simulink model "PMSM_to_BLDC_mod1"  (R2025b)
settings: Solver=FixedStepAuto  StartTime=0.0  StopTime=100  FixedStep=0.001  RelTol=1e-3
values from neighbouring files (symbols this model uses):
  B = 0.0025    [PMSM_to_BLDC_FOC.m]
  ctrl_reg1 = 0x02    [PMSM_to_BLDC_FOC.m]
  ctrl_reg2 = 0x03    [PMSM_to_BLDC_FOC.m]
  Damping_viscous = 0.00012    [PMSM_to_BLDC_FOC.m]
  J = 4.5e-5    (= 4.5e-05)    [PMSM_to_BLDC_FOC.m]
  Ki_Id = omg_clc * R_s    (= 464.72)    [PMSM_to_BLDC_FOC.m]
  Ki_Iq = omg_clc * R_s    (= 464.72)    [PMSM_to_BLDC_FOC.m]
  ki_speed = ((B *omg_cls * omg_cls)/(1.5*motor_polepairs*flux_linkage))    (= 157373.358662)    [PMSM_to_BLDC_FOC.m]
  Kp_Id = omg_clc * Ld    (= 22.608)    [PMSM_to_BLDC_FOC.m]
  Kp_Iq = omg_clc * Lq    (= 22.608)    [PMSM_to_BLDC_FOC.m]
  kp_speed = ((J*omg_cls)/(1.5*motor_polepairs*flux_linkage))    (= 2.25535068146)    [PMSM_to_BLDC_FOC.m]
  motor_polepairs = 7    [PMSM_to_BLDC_FOC.m]
  pwm_frequency = 20e3    (= 20000)    [PMSM_to_BLDC_FOC.m]
  read_reg = 1    [PMSM_to_BLDC_FOC.m]
  reg_ctrl_2 = ( bitshift(0,6) + bitshift(0,4) + bitshift(1,2) + bitshift(0,0))    [PMSM_to_BLDC_FOC.m]
  rps = x/6.28    (= 15.923566879)    [PMSM_to_BLDC_FOC.m]
  stat_reg1 = 0x00    [PMSM_to_BLDC_FOC.m]
  stat_reg2 = 0x01    [PMSM_to_BLDC_FOC.m]
  write_reg = 0    [PMSM_to_BLDC_FOC.m]
  x = 100    [PMSM_to_BLDC_FOC.m]
libraries: stm32blockslib x14, simulink x12, hdlsllib x10, nesl_utility x9, stm32f4xxblockslib x5, slpidlib x5, fl_lib x5, mcbeeMathTransformLib x3, ee_lib x3, mcbcontrolslib x1, mcbsensorlessestimatorlib x1, mcbplantlib x1
(part 1 of 2)
settings Model: STM32="{\"AnalogInput\":[{\"ID\":\"PMSM_to_BLDC_mod1:630\"},{\"ID\":\"PMSM_to_BLDC_mod1:900\"},{\"ID\":\"PMSM_to_BLDC_mod1:904\"}],\"PWMOutput\":{\"ID\":\"PMSM_to_BLDC_mod1:632\"},\"SPIControllerTransfer\":[{\"ID\":\"PMSM_to_BLDC_mod1:1052\"},{\"ID\":\"PMSM_to_BLDC_mod1:1051\"},{\"ID\":\"PMSM_to_BLDC_mod1:1149\"}],\"SPIControllerTransmit\":[{\"ID\":\"PMSM_to_BLDC_mod1:1060\"},{\"ID\":\"PMSM_to_BLDC_mod1:636:1184\"},{\"ID\":\"PMSM_to_BLDC_mod1:1221\"},{\"ID\":\"PMSM_to_BLDC_mod1:1178:1430\"},{\"ID\":\"PMSM_to_BLDC_mod1:1458\"},{\"ID\":\"PMSM_to_BLDC_mod1:1472\"},{\"ID\":\"PMSM_to_BLDC_mod1:1612\"},{\"ID\":\"PMSM_to_BLDC_mod1:1438\"},{\"ID\":\"PMSM_to_BLDC_mod1:1637\"},{\"ID\":\"PMSM_to_BLDC_mod1:1643\"}],\"DigitalPortWrite\":[{\"ID\":\"PMSM_to_BLDC_mod1:672\"},{\"ID\":\"PMSM_to_BLDC_mod1:1183\"}],\"SPIControllerReceive\":[{\"ID\":\"PMSM_to_BLDC_mod1:1178:1431\"},{\"ID\":\"PMSM_to_BLDC_mod1:1431\"},{\"ID\":\"PMSM_to_BLDC_mod1:1457\"},{\"ID\":\"PMSM_to_BLDC_mod1:1471\"},{\"ID\":\"PMSM_to_BLDC_mod1:1614\"},{\"ID\":\"PMSM_to_BLDC_mod1:1439\"},{\"ID\":\"PMSM_to_BLDC_mod1:1636\"},{\"ID\":\"PMSM_to_BLDC_mod1:1642\"}]}"  NumberOfSteps=5  Creator=Surinova  LastModifiedBy=Surinova
settings SolverCC: AutoInsertRateTranBlk=on
settings OptimizationCC: DefaultParameterBehavior=Inlined  EnhancedBackFolding=on  PassReuseOutputArgsAs=Individual arguments  ZeroExternalMemoryAtStartup=off  ZeroInternalMemoryAtStartup=off  MaxStackSize=512  OptimizeBlockOrder=speed  DifferentSizesBufferReuse=on  OptimizationCustomize=off  EfficientTunableParamExpr=on
settings DebuggingCC: ParameterTunabilityLossMsg=error
settings HardwareCC: ProdBitPerPointer=32.0  ProdBitPerSizeT=32.0  ProdBitPerPtrDiffT=32.0  ProdLargestAtomicInteger=Long  ProdLargestAtomicFloat=Double  ProdWordSize=32.0  ProdLongLongMode=on  ProdHWDeviceType=ARM Compatible->ARM Cortex-M
settings SFSimCC: SimCustomHeaderCode="\"C:\\Users\\Surinova\\OneDrive - Surinova Pvt Ltd\\Documents\\Github\\MatLab_FOC_model\\FOC_model_1\\SPI_code.h\""  SimUserSources="\"C:\\Users\\Surinova\\OneDrive - Surinova Pvt Ltd\\Documents\\Github\\MatLab_FOC_model\\FOC_model_1\\SPI_code.c\""  MATLABDynamicMemAlloc=off
settings RTWCC: SystemTargetFile=ert.tlc  HardwareBoard=STM32F4xx Based  TemplateMakefile=ert_default_tmf  GenerateReport=on  Toolchain=GNU Tools for ARM Embedded Processors  LaunchReport=on  Description=Embedded Coder
settings RTWCC: CustomHeaderCode=|
  | #include "main.h"
  | #include "SPI_code.h"
  | #include "spi.h"
  | #include "dma.h"
  | #include "gpio.h"
  | #include "tim.h"
  | #include "adc.h"
  | #include "usart.h"
settings RTWCC: CustomInclude=|
  | "C:\Users\Surinova\OneDrive - Surinova Pvt Ltd\Documents\Github\MatLab_FOC_model\FOC_model_1"
  | "C:\Users\Surinova\OneDrive - Surinova Pvt Ltd\Documents\Github\MatLab_FOC_model\F405_PMSM_Mod1\Core\Inc"
  | "C:\Users\Surinova\OneDrive - Surinova Pvt Ltd\Documents\Github\MatLab_FOC_model\F405_PMSM_Mod1\Drivers\STM32F4xx_HAL_Driver\Inc"
  | "C:\Users\Surinova\OneDrive - Surinova Pvt Ltd\Documents\Github\MatLab_FOC_model\F405_PMSM_Mod1\Drivers\CMSIS\Include"
  | "C:\Users\Surinova\OneDrive - Surinova Pvt Ltd\Documents\Github\MatLab_FOC_model\F405_PMSM_Mod1\Drivers\CMSIS\Device\ST\STM32F4xx\Include"
settings RTWCC: CustomSource=|
  | SPI_code.c
  | "C:\Users\Surinova\OneDrive - Surinova Pvt Ltd\Documents\Github\MatLab_FOC_model\F405_PMSM_Mod1\Drivers\STM32F4xx_HAL_Driver\Src\stm32f4xx_hal_spi.c"
  | "C:\Users\Surinova\OneDrive - Surinova Pvt Ltd\Documents\Github\MatLab_FOC_model\F405_PMSM_Mod1\Core\Src\spi.c"
  | "C:\Users\Surinova\OneDrive - Surinova Pvt Ltd\Documents\Github\MatLab_FOC_model\F405_PMSM_Mod1\Core\Src\adc.c"
  | "C:\Users\Surinova\OneDrive - Surinova Pvt Ltd\Documents\Github\MatLab_FOC_model\F405_PMSM_Mod1\Core\Src\dma.c"
  | "C:\Users\Surinova\OneDrive - Surinova Pvt Ltd\Documents\Github\MatLab_FOC_model\F405_PMSM_Mod1\Core\Src\gpio.c"
  | "C:\Users\Surinova\OneDrive - Surinova Pvt Ltd\Documents\Github\MatLab_FOC_model\F405_PMSM_Mod1\Core\Src\tim.c"
  | "C:\Users\Surinova\OneDrive - Surinova Pvt Ltd\Documents\Github\MatLab_FOC_model\F405_PMSM_Mod1\Core\Src\usart.c"
settings CodeAppCC: ForceParamTrailComments=on  IgnoreCustomStorageClasses=off  OperatorAnnotations=on  SimulinkDataObjDesc=on  SFDataObjDesc=on  InsertBlockDesc=on
settings ERTTargetCC: ExtModeTransport=3.0  ExtModeStaticAlloc=on  ExtModeStaticAllocSize=2048.0  ExtModeMexFile=ext_xcp  ExtModeIntrfLevel=Level2 - Open  TargetLangStandard=C99 (ISO)  CodeReplacementLibrary=ARM Cortex-M  SupportContinuousTime=on

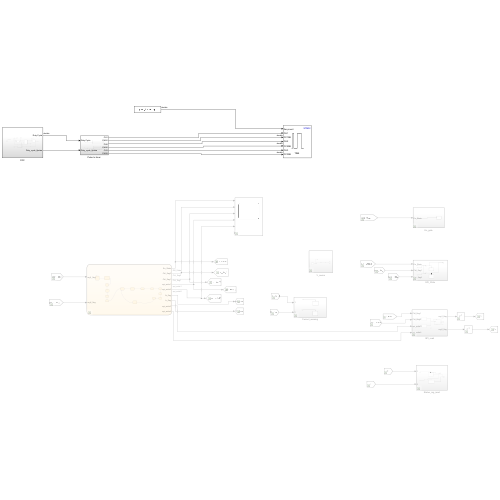
[thumbnail: Simulink's stored preview of the top-level diagram]
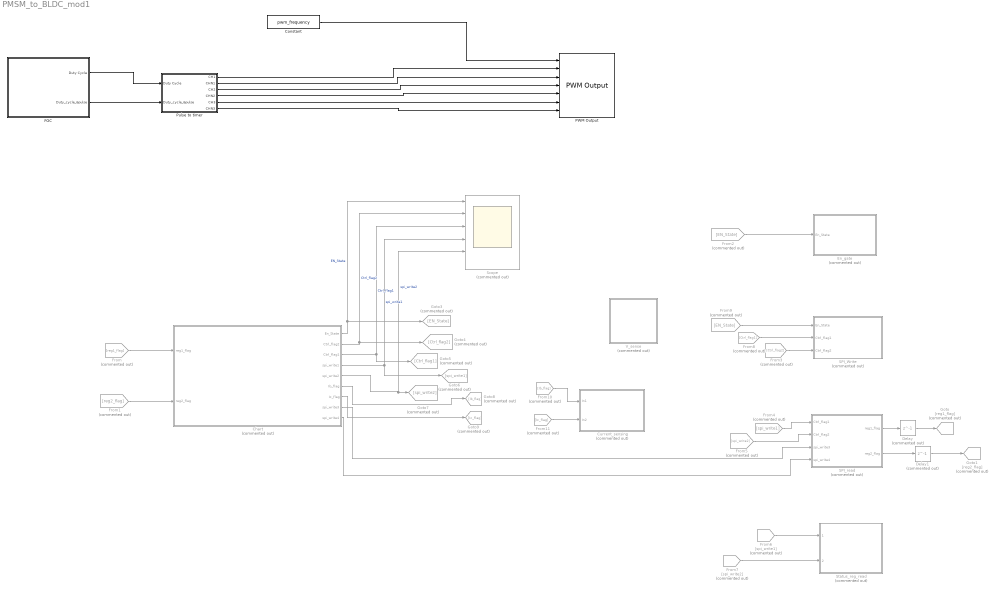
== system PMSM_to_BLDC_mod1 ==
  Chart : Stateflow chart  Commented=on  TreatAsAtomicUnit=on
  Constant : Constant  Value=pwm_frequency
  Current_sensing : Subsystem  Commented=on
  Delay : Delay  Commented=on  DelayLength=1  InputProcessing=Columns as channels (frame based)
  Delay1 : Delay  Commented=on  DelayLength=1  InputProcessing=Columns as channels (frame based)
  En_gate : Subsystem  Commented=on
  FOC : Subsystem
  From : From  Commented=on  GotoTag=reg1_flag
  From1 : From  Commented=on  GotoTag=reg2_flag
  From10 : From  Commented=on  GotoTag=Ib_flag
  From11 : From  Commented=on  GotoTag=Ic_flag
  From2 : From  Commented=on  GotoTag=EN_State
  From3 : From  Commented=on  GotoTag=Ctrl_flag2
  From4 : From  Commented=on  GotoTag=spi_write1
  From5 : From  Commented=on  GotoTag=spi_write2
  From6 : From  Commented=on  GotoTag=spi_write1
  From7 : From  Commented=on  GotoTag=spi_write2
  From8 : From  Commented=on  GotoTag=Ctrl_flag1
  From9 : From  Commented=on  GotoTag=EN_State
  Goto : Goto  Commented=on  GotoTag=reg1_flag
  Goto1 : Goto  Commented=on  GotoTag=reg2_flag
  Goto3 : Goto  Commented=on  GotoTag=EN_State
  Goto4 : Goto  Commented=on  GotoTag=Ctrl_flag2
  Goto5 : Goto  Commented=on  GotoTag=Ctrl_flag1
  Goto6 : Goto  Commented=on  GotoTag=spi_write1
  Goto7 : Goto  Commented=on  GotoTag=spi_write2
  Goto8 : Goto  Commented=on  GotoTag=Ib_flag
  Goto9 : Goto  Commented=on  GotoTag=Ic_flag
  PWM Output : stm32f4xxblockslib/PWM Output  ProcessorFamily=STM32F4  TimerModule=TIM8  DutycycleUnits=Percentage  EnableChannel1=on  EnableCaptureCompare1Input=off  EnableCaptureCompare1ComplementaryInput=on  EnableOutputCompare1ModeInput=off  EnableChannel2=on  EnableCaptureCompare2Input=off  EnableCaptureCompare2ComplementaryInput=on  EnableOutputCompare2ModeInput=off  EnableChannel3=on  EnableCaptureCompare3Input=off  EnableCaptureCompare3ComplementaryInput=on  EnableOutputCompare3ModeInput=off  EnableChannel4=off  EnableCaptureCompare4Input=off  EnableCaptureCompare4ComplementaryInput=off  EnableOutputCompare4ModeInput=off  EnableChannel5=off  EnableCaptureCompare5Input=off  EnableOutputCompare5ModeInput=off  EnableChannel6=off  EnableCaptureCompare6Input=off  EnableOutputCompare6ModeInput=off  EnableCounterInput=off  EnableMainOutputInput=off  EnableFrequencyInput=on  SetRCAfterCE=on  OutputDirection=off  OutputMainOutputEnableStatus=off  SampleTime=0.1  EnableSimPort=off  EnableUpdateEvent=off  EnableCaptureCompare1Event=off  EnableCaptureCompare2Event=off  EnableCaptureCompare3Event=off  EnableCaptureCompare4Event=off  EnableTriggerEvent=off  EnableBreakEvent=off  EnableBreakEvent2=off  hoistedMaskSrc=ECSoC/ECSimCodegen/PWM Output
  "Pulse to timer " : Subsystem
  SPI_Write : Subsystem  Commented=on
  SPI_read : Subsystem  Commented=on
  Scope : Scope  Commented=on  NumInputPorts=6
      settings: ActiveDisplayYMinimum=-0.011045533032348887  ActiveDisplayYMaximum=0.023895922034976431  DataLoggingVariableName=ScopeData17
  Status_reg_read : Subsystem  Commented=on
  V_sense : Subsystem  Commented=on
  wires:
  Constant/1 -> PWM Output/1
  FOC/1(Duty Cycle) -> "Pulse to timer "/1(Duty Cycle)
  SPI_read/1(reg1_flag) -> Delay/1
  SPI_read/2(reg2_flag) -> Delay1/1
  From/1 -> Chart/1(reg1_flag)
  From1/1 -> Chart/2(reg2_flag)
  Chart/1(En_State) -> Scope/1, Goto3/1  "EN_State"
  Chart/2(Ctrl_flag2) -> Goto4/1, Scope/2  "Ctrl_flag2"
  Chart/3(Ctrl_flag1) -> Goto5/1, Scope/3  "Ctrl_flag1"
  Chart/4(spi_write1) -> Goto6/1, Scope/4  "spi_write1"
  Chart/5(spi_write2) -> Goto7/1, Scope/5  "spi_write2"
  Chart/6(Ib_flag) -> Goto8/1
  Chart/7(Ic_flag) -> Goto9/1
  From2/1 -> En_gate/1(En_State)
  From9/1 -> SPI_Write/1(En_State)
  From8/1 -> SPI_Write/2(Ctrl_flag1)
  From4/1 -> SPI_read/1(Ctrl_flag1)
  From5/1 -> SPI_read/2(Ctrl_flag2)
  From6/1 -> Status_reg_read/1(1)
  From7/1 -> Status_reg_read/2(2)
  From10/1 -> Current_sensing/1(In1)
  From11/1 -> Current_sensing/2(In2)
  From3/1 -> SPI_Write/3(Ctrl_flag2)
  Chart/8(spi_write3) -> SPI_read/3(spi_write3)
  Chart/9(spi_write4) -> SPI_read/4(spi_write4)
  Delay/1 -> Goto/1
  Delay1/1 -> Goto1/1
  FOC/2(Duty_cycle_6pulse) -> "Pulse to timer "/2(Duty_cycle_6pulse)
  "Pulse to timer "/1(CH1) -> PWM Output/2
  "Pulse to timer "/2(CHN1) -> PWM Output/3
  "Pulse to timer "/3(CH2) -> PWM Output/4
  "Pulse to timer "/4(CHN2) -> PWM Output/5
  "Pulse to timer "/5(CH3) -> PWM Output/6
  "Pulse to timer "/6(CHN3) -> PWM Output/7

== system PMSM_to_BLDC_mod1/Current_sensing ==
  In1 : Inport
  In2 : Inport  Port=2
  Subsystem : Subsystem
  Subsystem1 : Subsystem
  wires:
  In1/1 -> Subsystem/Enable
  In2/1 -> Subsystem1/Enable

== system PMSM_to_BLDC_mod1/En_gate ==
  En_State : Inport
  Digital Port Write : stm32f4xxblockslib/Digital Port Write  PortName=GPIOB  PinNumber=12  ReadOperation=off  IOAsArray=on  EnableSimPort=off  hoistedMaskSrc=ECSoC/ECSimCodegen/Digital Port Write
  wires:
  En_State/1 -> Digital Port Write/1

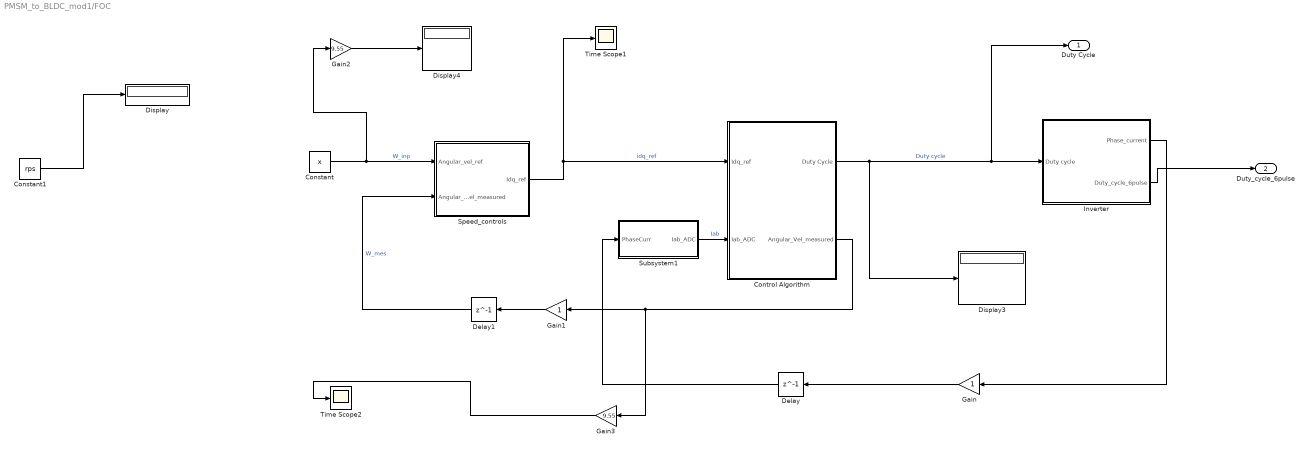
== system PMSM_to_BLDC_mod1/FOC ==
  Constant : Constant  Value=x
  Constant1 : Constant  Value=rps
  "Control Algorithm " : Subsystem
  Delay : Delay  DelayLength=1
  Delay1 : Delay  DelayLength=1
  Display : Display
  Display3 : Display
  Display4 : Display
  Gain : Gain
  Gain1 : Gain
  Gain2 : Gain  Gain=9.55
  Gain3 : Gain  Gain=9.55
  Inverter : Subsystem
  Speed_controls : Subsystem
  Subsystem1 : Subsystem
  Time Scope1 : Scope
      settings: TimeUnits=Metric (based on Time Span)  ActiveDisplayYMinimum=-1278.396312713623  ActiveDisplayYMaximum=607.25992965698242  YLabel=Amplitude
  Time Scope2 : Scope
      settings: TimeUnits=Metric (based on Time Span)  ActiveDisplayYMinimum=-2551.3535904439232  ActiveDisplayYMaximum=7986.0366937033405  YLabel=Amplitude  DataLoggingVariableName=ScopeData5
  Duty Cycle : Outport
  Duty_cycle_6pulse : Outport  Port=2
  wires:
  Delay1/1 -> Speed_controls/2(Angular_vel_measured)  "W_mes"
  Subsystem1/1(Iab_ADC) -> "Control Algorithm "/2(Iab_ADC)  "Iab"
  Gain3/1 -> Time Scope2/1
  Constant/1 -> Gain2/1, Speed_controls/1(Angular_vel_ref)  "W_inp"
  Gain/1 -> Delay/1
  "Control Algorithm "/2(Angular_Vel_measured) -> Gain1/1, Gain3/1
  Gain2/1 -> Display4/1
  "Control Algorithm "/1(Duty Cycle) -> Duty Cycle/1, Inverter/1(Duty cycle), Display3/1  "Duty cycle"
  Constant1/1 -> Display/1
  Speed_controls/1(Idq_ref) -> Time Scope1/1, "Control Algorithm "/1(Idq_ref)  "idq_ref"
  Gain1/1 -> Delay1/1
  Inverter/1(Phase_current) -> Gain/1
  Delay/1 -> Subsystem1/1(PhaseCurr)
  Inverter/2(Duty_cycle_6pulse) -> Duty_cycle_6pulse/1

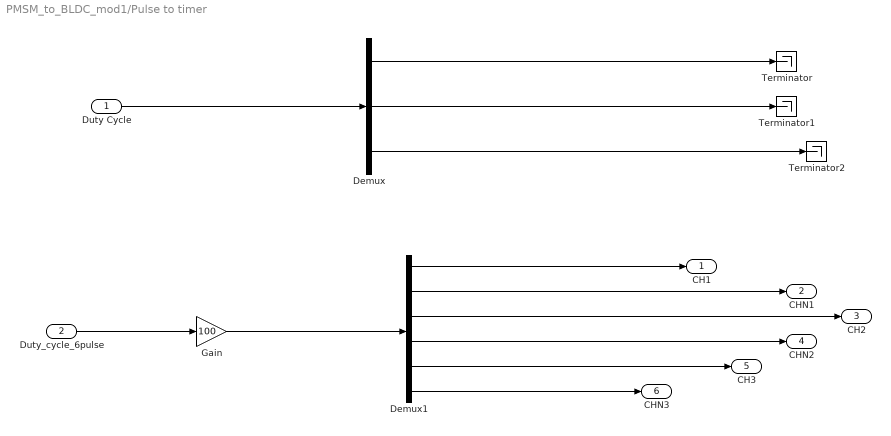
== system PMSM_to_BLDC_mod1/Pulse to timer  ==
  Duty Cycle : Inport
  Duty_cycle_6pulse : Inport  Port=2
  Demux : Demux  Outputs=3
  Demux1 : Demux  Outputs=6
  Gain : Gain  Gain=100
  Terminator : Terminator
  Terminator1 : Terminator
  Terminator2 : Terminator
  CH1 : Outport
  CHN1 : Outport  Port=2
  CH2 : Outport  Port=3
  CHN2 : Outport  Port=4
  CH3 : Outport  Port=5
  CHN3 : Outport  Port=6
  wires:
  Duty Cycle/1 -> Demux/1
  Demux/3 -> Terminator2/1
  Demux/1 -> Terminator/1
  Demux/2 -> Terminator1/1
  Duty_cycle_6pulse/1 -> Gain/1
  Demux1/1 -> CH1/1
  Demux1/2 -> CHN1/1
  Demux1/3 -> CH2/1
  Demux1/4 -> CHN2/1
  Demux1/5 -> CH3/1
  Demux1/6 -> CHN3/1
  Gain/1 -> Demux1/1

== system PMSM_to_BLDC_mod1/SPI_Write ==
  En_State : Inport
  Ctrl_flag1 : Inport  Port=2
  Ctrl_flag2 : Inport  Port=3
  AND : Logic  IconShape=distinctive  AllPortsSameDT=off  OutDataTypeStr=boolean
  AND1 : Logic  IconShape=distinctive  AllPortsSameDT=off  OutDataTypeStr=boolean
  Control_Reg2 : Subsystem
  Ctrl_Reg_1 : Subsystem  ReferencedSubsystem=Ctrl_Reg_1
  Scope : Scope  NumInputPorts=2
      settings: ActiveDisplayYMinimum=-0.12499999999999997  ActiveDisplayYMaximum=1.125  DataLoggingVariableName=ScopeData18
  wires:
  Ctrl_flag1/1 -> AND/2
  En_State/1 -> AND1/1, AND/1
  AND/1 -> Scope/1, Ctrl_Reg_1/Enable
  AND1/1 -> Control_Reg2/Enable, Scope/2
  Ctrl_flag2/1 -> AND1/2

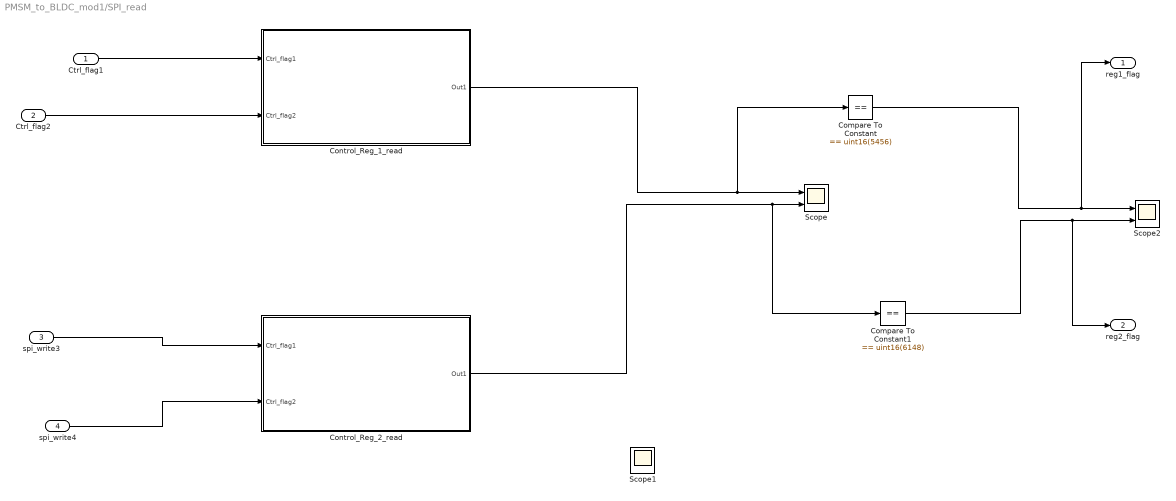
== system PMSM_to_BLDC_mod1/SPI_read ==
  Ctrl_flag1 : Inport
  Ctrl_flag2 : Inport  Port=2
  spi_write3 : Inport  Port=3
  spi_write4 : Inport  Port=4
  Compare To Constant : simulink/Logic and Bit Operations/Compare To Constant  relop===  const=uint16(5456)  OutDataTypeStr=boolean
  Compare To Constant1 : simulink/Logic and Bit Operations/Compare To Constant  relop===  const=uint16(6148)  OutDataTypeStr=boolean
  Control_Reg_1_read : Subsystem
  Control_Reg_2_read : Subsystem
  Scope : Scope  NumInputPorts=2
      settings: ActiveDisplayYMinimum=-4607.9999999999991  ActiveDisplayYMaximum=41472  DataLoggingVariableName=ScopeData13
  Scope1 : Scope  NumInputPorts=2
      settings: ActiveDisplayYMinimum=-0.082255061291701556  ActiveDisplayYMaximum=0.18007764693489475  DataLoggingVariableName=ScopeData21
  Scope2 : Scope  NumInputPorts=2
      settings: ActiveDisplayYMinimum=-0.12499999999999997  ActiveDisplayYMaximum=1.125  DataLoggingVariableName=ScopeData15
  reg1_flag : Outport
  reg2_flag : Outport  Port=2
  wires:
  Compare To Constant/1 -> reg1_flag/1, Scope2/1
  Ctrl_flag1/1 -> Control_Reg_1_read/1(Ctrl_flag1)
  Ctrl_flag2/1 -> Control_Reg_1_read/2(Ctrl_flag2)
  spi_write3/1 -> Control_Reg_2_read/1(Ctrl_flag1)
  spi_write4/1 -> Control_Reg_2_read/2(Ctrl_flag2)
  Control_Reg_1_read/1(Out1) -> Compare To Constant/1, Scope/1
  Control_Reg_2_read/1(Out1) -> Compare To Constant1/1, Scope/2
  Compare To Constant1/1 -> reg2_flag/1, Scope2/2

== system PMSM_to_BLDC_mod1/Status_reg_read ==
  1 : Inport
  2 : Inport  Port=2
  Scope : Scope  NumInputPorts=2
      settings: ActiveDisplayYMinimum=-1.2810969274237476  ActiveDisplayYMaximum=1.2714661975762531  DataLoggingVariableName=ScopeData14
  Scope1 : Scope  NumInputPorts=2
      settings: ActiveDisplayYMinimum=-1.7236670282456201  ActiveDisplayYMaximum=2.8116607909152096  DataLoggingVariableName=ScopeData16
  Status_Reg1_read : Subsystem
  Status_Reg_2_read : Subsystem
  wires:
  1/1 -> Scope1/1, Status_Reg1_read/Enable
  Status_Reg1_read/1(Out1) -> Scope/2
  Status_Reg_2_read/1(Out1) -> Scope/1
  2/1 -> Scope1/2, Status_Reg_2_read/Enable

== system PMSM_to_BLDC_mod1/V_sense ==
  Analog to Digital Converter1 : stm32f4xxblockslib/Analog to Digital Converter  ADCModule=ADC1  ConversionGroup=Regular  TriggerMode=Trigger and read  NumberOfConversions=1  EnableBufferConv=off  BufferLength=1  OutputStatus=off  SampleTime=0.1  EnableSimPort=off  hoistedMaskSrc=ECSoC/ECSimCodegen/Analog to Digital Converter
  Data Type Conversion : DataTypeConversion  OutDataTypeStr=double  SaturateOnIntegerOverflow=off  RndMeth=Floor
  Display : Display
  Gain : Gain  Gain=50/3200
  Scope : Scope
      settings: ActiveDisplayYMinimum=1998.2131563180828  ActiveDisplayYMaximum=2530.7206563180825  DataLoggingVariableName=ScopeData12
  wires:
  Analog to Digital Converter1/1 -> Scope/1, Data Type Conversion/1
  Gain/1 -> Display/1
  Data Type Conversion/1 -> Gain/1

== system PMSM_to_BLDC_mod1/Current_sensing/Subsystem ==
  Enable : EnablePort
  Analog to Digital Converter1 : stm32f4xxblockslib/Analog to Digital Converter  ADCModule=ADC2  ConversionGroup=Regular  TriggerMode=Trigger and read  NumberOfConversions=1  EnableBufferConv=off  BufferLength=1  OutputStatus=off  SampleTime=0.1  EnableSimPort=off  hoistedMaskSrc=ECSoC/ECSimCodegen/Analog to Digital Converter
  Data Type Conversion : DataTypeConversion  OutDataTypeStr=double  SaturateOnIntegerOverflow=off  RndMeth=Floor
  Display1 : Display
  Gain : Gain  Gain=100/4095
  wires:
  Gain/1 -> Display1/1
  Analog to Digital Converter1/1 -> Data Type Conversion/1
  Data Type Conversion/1 -> Gain/1

== system PMSM_to_BLDC_mod1/Current_sensing/Subsystem1 ==
  Enable : EnablePort
  Analog to Digital Converter2 : stm32f4xxblockslib/Analog to Digital Converter  ADCModule=ADC3  ConversionGroup=Regular  TriggerMode=Trigger and read  NumberOfConversions=1  EnableBufferConv=off  BufferLength=1  OutputStatus=off  SampleTime=0.1  EnableSimPort=off  hoistedMaskSrc=ECSoC/ECSimCodegen/Analog to Digital Converter
  Data Type Conversion1 : DataTypeConversion  OutDataTypeStr=double  SaturateOnIntegerOverflow=off  RndMeth=Floor
  Display2 : Display
  Gain1 : Gain  Gain=100/4095
  wires:
  Gain1/1 -> Display2/1
  Analog to Digital Converter2/1 -> Data Type Conversion1/1
  Data Type Conversion1/1 -> Gain1/1

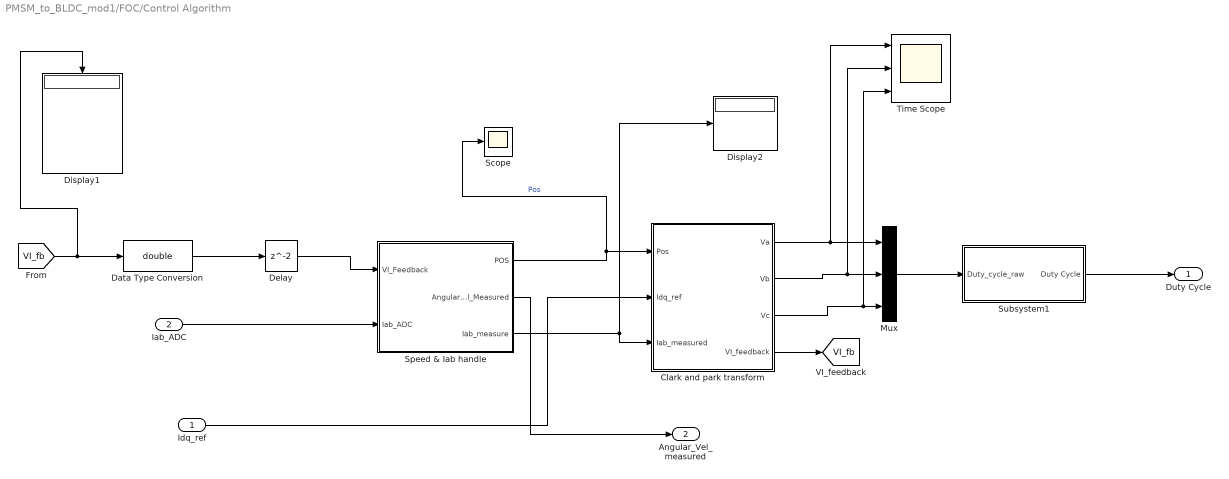
== system PMSM_to_BLDC_mod1/FOC/Control Algorithm  ==
  Idq_ref : Inport
  Iab_ADC : Inport  Port=2
  Clark and park transform : Subsystem
  Data Type Conversion : DataTypeConversion  OutDataTypeStr=double  SaturateOnIntegerOverflow=off  RndMeth=Floor
  Delay : Delay
  Display1 : Display
  Display2 : Display
  Mux : Mux  Inputs=3
  Scope : Scope
      settings: ActiveDisplayYMinimum=-2.9858848726720835  ActiveDisplayYMaximum=10.141823403799465  DataLoggingVariableName=ScopeData4
  Speed & Iab handle : Subsystem
  Subsystem1 : Subsystem
  Time Scope : Scope  NumInputPorts=3
      settings: TimeUnits=Metric (based on Time Span)  ActiveDisplayYMinimum=-4.3489349004753368  ActiveDisplayYMaximum=5.723501707770442  YLabel=Amplitude  DataLoggingVariableName=ScopeData2
  Duty Cycle : Outport
  Angular_Vel_measured : Outport  Port=2
  tag scope: VI_fb=global
  wires:
  Clark and park transform/4(VI_feedback) -> [VI_fb]
  Clark and park transform/3(Vc) -> Mux/3, Time Scope/3
  [VI_fb] -> Display1/1, Data Type Conversion/1
  Mux/1 -> Subsystem1/1(Duty_cycle_raw)
  Iab_ADC/1 -> Speed & Iab handle/2(Iab_ADC)
  Speed & Iab handle/3(Iab_measure) -> Clark and park transform/3(Iab_measured), Display2/1
  Clark and park transform/2(Vb) -> Mux/2, Time Scope/2
  Clark and park transform/1(Va) -> Time Scope/1, Mux/1
  Speed & Iab handle/2(Angular_Vel_Measured) -> Angular_Vel_measured/1
  Idq_ref/1 -> Clark and park transform/2(Idq_ref)
  Delay/1 -> Speed & Iab handle/1(VI_Feedback)
  Data Type Conversion/1 -> Delay/1
  Speed & Iab handle/1(POS) -> Scope/1, Clark and park transform/1(Pos)  "Pos"
  Subsystem1/1(Duty Cycle) -> Duty Cycle/1

== system PMSM_to_BLDC_mod1/FOC/Inverter ==
  Duty cycle : Inport
  Simulation : Subsystem
  Subsystem2 : Subsystem
  Phase_current : Outport
  Duty_cycle_6pulse : Outport  Port=2
  wires:
  Duty cycle/1 -> Simulation/2(Duty_cycle), Subsystem2/1(Duty cycle)
  Simulation/1(Phase_current) -> Phase_current/1
  Subsystem2/1(Duty_cycle_6pulse) -> Duty_cycle_6pulse/1, Simulation/1(Gate_pulse)  "Gate_pulse"

== system PMSM_to_BLDC_mod1/FOC/Speed_controls ==
  Angular_vel_ref : Inport
  Angular_vel_measured : Inport  Port=2
  Add : Sum  Inputs=+-
  Constant : Constant  Value=0
  Display : Display
  Mux : Mux  Inputs=2
  Saturation : Saturate  UpperLimit=600  LowerLimit=-600
  Scope : Scope
      settings: ActiveDisplayYMinimum=-1  ActiveDisplayYMaximum=1  DataLoggingVariableName=ScopeData3
  Speed Control : Subsystem
  Idq_ref : Outport  PortDimensions=2
  wires:
  Angular_vel_measured/1 -> Saturation/1
  Add/1 -> Display/1, Speed Control/1(u)
  Mux/1 -> Idq_ref/1
  Speed Control/1(Iq_ref) -> Scope/1, Mux/2
  Constant/1 -> Mux/1
  Angular_vel_ref/1 -> Add/1
  Saturation/1 -> Add/2

== system PMSM_to_BLDC_mod1/FOC/Subsystem1 ==
  PhaseCurr : Inport
  Iab_ADC : Outport
  wires:
  PhaseCurr/1 -> Iab_ADC/1

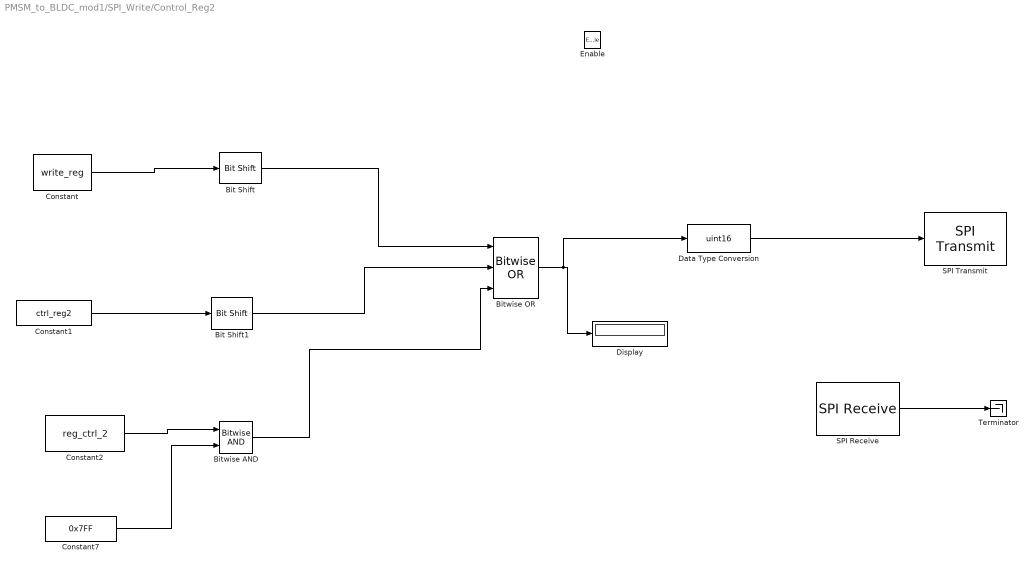
== system PMSM_to_BLDC_mod1/SPI_Write/Control_Reg2 ==
  Enable : EnablePort  StatesWhenEnabling=reset
  Bit Shift : hdlsllib/Logic and Bit Operations/Bit Shift  mode=Shift Left Logical  N=15
  Bit Shift1 : hdlsllib/Logic and Bit Operations/Bit Shift  mode=Shift Left Logical  N=11
  Bitwise AND : simulink/Logic and Bit Operations/Bitwise Operator  logicop=AND  UseBitMask=off  NumInputPorts=2  BitMask=bin2dec('11011001')  BitMaskRealWorld=Stored Integer
      settings: LibrarySourceBlock=|
      | simulink/Quick Insert/Logic and Bit
      | Operations/Bitwise AND
  Bitwise OR : simulink/Logic and Bit Operations/Bitwise Operator  logicop=OR  UseBitMask=off  NumInputPorts=3  BitMask=bin2dec('11011001')  BitMaskRealWorld=Stored Integer
      settings: LibrarySourceBlock=|
      | simulink/Quick Insert/Logic and Bit
      | Operations/Bitwise OR
  Constant : Constant  Value=write_reg  OutDataTypeStr=uint16
  Constant1 : Constant  Value=ctrl_reg2  OutDataTypeStr=uint16
  Constant2 : Constant  Value=reg_ctrl_2  OutDataTypeStr=uint16
  Constant7 : Constant  Value=0x7FF  OutDataTypeStr=uint16
  Data Type Conversion : DataTypeConversion  OutDataTypeStr=uint16  SaturateOnIntegerOverflow=off  RndMeth=Floor
  Display : Display
      settings: Format=hex (Stored Integer)
  SPI Receive : stm32blockslib/SPI Receive  SPIModuleSelect=SPI3  ClockPolarity=Low  ClockPhase=2 Edge  SPIModule=uint32(0)  Mode=Master  BusSpeed=uint32(1000000)  FirstBitToTransfer=Most significant bit (MSB)  ClockMode=0  BlockFunction=Read  EnableRegisterAddress=on  RegisterAddress=0  OutputDataType=uint8  OutputDataLength=16  OutputStatus=off  BlockingMode=on  Timeout=0.001  SampleTime=-1  DataBits=16  UseCustomSSPin=Explicit GPIO calls  ActiveLowSSPin=Active low  Port_Select=GPIOC  Pin=14
      settings: LibrarySourceBlock=stm32f4xxblockslib/SPI Receive
  SPI Transmit : stm32blockslib/SPI Transmit  SPIModuleSelect=SPI3  ClockPolarity=Low  ClockPhase=2 Edge  SPIModule=uint32(0)  Mode=Master  BusSpeed=uint32(1000000)  FirstBitToTransfer=Most significant bit (MSB)  ClockMode=0  BlockFunction=Write  EnableRegisterAddress=on  RegisterAddress=0  OutputDataType=uint8  OutputDataLength=1  OutputStatus=off  BlockingMode=on  Timeout=1  DataBits=16  UseCustomSSPin=Explicit GPIO calls  ActiveLowSSPin=Active low  Port_Select=GPIOC  Pin=14
      settings: LibrarySourceBlock=stm32f4xxblockslib/SPI Transmit
  Terminator : Terminator
  wires:
  Constant/1 -> Bit Shift/1
  Bit Shift/1 -> Bitwise OR/1
  Bit Shift1/1 -> Bitwise OR/2
  Constant2/1 -> Bitwise AND/1
  Constant7/1 -> Bitwise AND/2
  Bitwise AND/1 -> Bitwise OR/3
  Bitwise OR/1 -> Data Type Conversion/1, Display/1
  Data Type Conversion/1 -> SPI Transmit/1
  Constant1/1 -> Bit Shift1/1
  SPI Receive/1 -> Terminator/1

== system PMSM_to_BLDC_mod1/SPI_read/Control_Reg_1_read ==
  Ctrl_flag1 : Inport
  Ctrl_flag2 : Inport  Port=2
  Subsystem : Subsystem
  Subsystem1 : Subsystem
  Out1 : Outport  OutputWhenDisabled=reset  InitialOutput=[0]
  wires:
  Ctrl_flag1/1 -> Subsystem/Enable
  Ctrl_flag2/1 -> Subsystem1/Enable
  Subsystem1/1(Out1) -> Out1/1

== system PMSM_to_BLDC_mod1/SPI_read/Control_Reg_2_read ==
  Ctrl_flag1 : Inport
  Ctrl_flag2 : Inport  Port=2
  Subsystem : Subsystem
  Subsystem1 : Subsystem
  Out1 : Outport
  wires:
  Ctrl_flag1/1 -> Subsystem/Enable
  Ctrl_flag2/1 -> Subsystem1/Enable
  Subsystem1/1(Out1) -> Out1/1

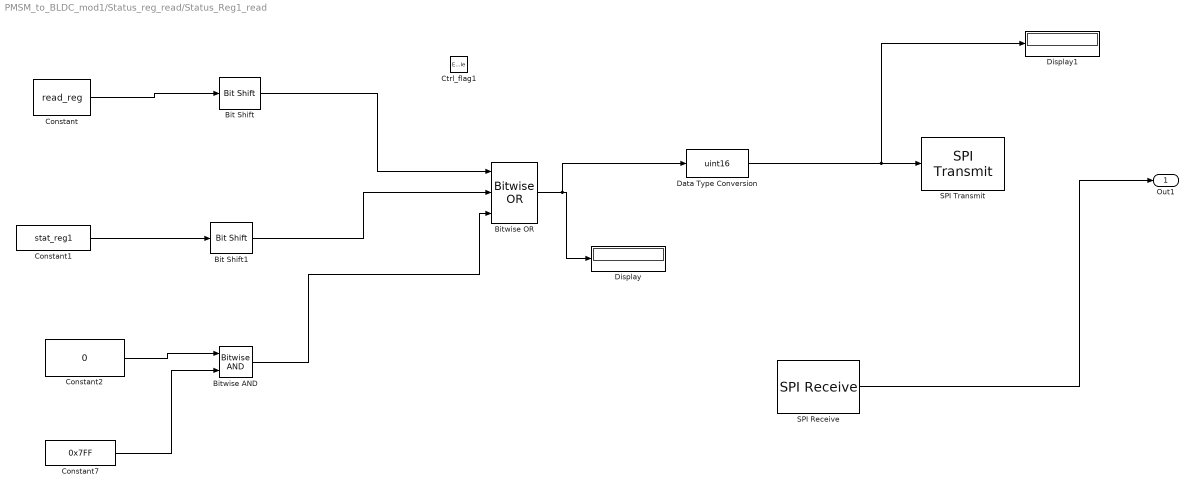
== system PMSM_to_BLDC_mod1/Status_reg_read/Status_Reg1_read ==
  Ctrl_flag1 : EnablePort  StatesWhenEnabling=reset
  Bit Shift : hdlsllib/Logic and Bit Operations/Bit Shift  mode=Shift Left Logical  N=15
  Bit Shift1 : hdlsllib/Logic and Bit Operations/Bit Shift  mode=Shift Left Logical  N=11
  Bitwise AND : simulink/Logic and Bit Operations/Bitwise Operator  logicop=AND  UseBitMask=off  NumInputPorts=2  BitMask=bin2dec('11011001')  BitMaskRealWorld=Stored Integer
      settings: LibrarySourceBlock=|
      | simulink/Quick Insert/Logic and Bit
      | Operations/Bitwise AND
  Bitwise OR : simulink/Logic and Bit Operations/Bitwise Operator  logicop=OR  UseBitMask=off  NumInputPorts=3  BitMask=bin2dec('11011001')  BitMaskRealWorld=Stored Integer
      settings: LibrarySourceBlock=|
      | simulink/Quick Insert/Logic and Bit
      | Operations/Bitwise OR
  Constant : Constant  Value=read_reg  OutDataTypeStr=uint16
  Constant1 : Constant  Value=stat_reg1  OutDataTypeStr=uint16
  Constant2 : Constant  Value=0  OutDataTypeStr=uint16
  Constant7 : Constant  Value=0x7FF  OutDataTypeStr=uint16
  Data Type Conversion : DataTypeConversion  OutDataTypeStr=uint16  SaturateOnIntegerOverflow=off  RndMeth=Floor
  Display : Display
      settings: Format=hex (Stored Integer)
  Display1 : Display
      settings: Format=hex (Stored Integer)
  SPI Receive : stm32blockslib/SPI Receive  SPIModuleSelect=SPI3  ClockPolarity=Low  ClockPhase=2 Edge  SPIModule=uint32(0)  Mode=Master  BusSpeed=uint32(1000000)  FirstBitToTransfer=Most significant bit (MSB)  ClockMode=0  BlockFunction=Read  EnableRegisterAddress=on  RegisterAddress=0  OutputDataType=uint8  OutputDataLength=15  OutputStatus=off  BlockingMode=on  Timeout=0.001  SampleTime=-1  DataBits=16  UseCustomSSPin=Explicit GPIO calls  ActiveLowSSPin=Active low  Port_Select=GPIOC  Pin=14
      settings: LibrarySourceBlock=stm32f4xxblockslib/SPI Receive
  SPI Transmit : stm32blockslib/SPI Transmit  SPIModuleSelect=SPI3  ClockPolarity=Low  ClockPhase=2 Edge  SPIModule=uint32(0)  Mode=Master  BusSpeed=uint32(1000000)  FirstBitToTransfer=Most significant bit (MSB)  ClockMode=0  BlockFunction=Write  EnableRegisterAddress=on  RegisterAddress=0  OutputDataType=uint8  OutputDataLength=1  OutputStatus=off  BlockingMode=on  Timeout=0.001  DataBits=16  UseCustomSSPin=Explicit GPIO calls  ActiveLowSSPin=Active low  Port_Select=GPIOC  Pin=14
      settings: LibrarySourceBlock=stm32f4xxblockslib/SPI Transmit
  Out1 : Outport  OutputWhenDisabled=reset  InitialOutput=[0]
  wires:
  Constant/1 -> Bit Shift/1
  Bit Shift/1 -> Bitwise OR/1
  Bit Shift1/1 -> Bitwise OR/2
  Constant2/1 -> Bitwise AND/1
  Constant7/1 -> Bitwise AND/2
  Bitwise AND/1 -> Bitwise OR/3
  Bitwise OR/1 -> Data Type Conversion/1, Display/1
  Constant1/1 -> Bit Shift1/1
  Data Type Conversion/1 -> SPI Transmit/1, Display1/1
  SPI Receive/1 -> Out1/1

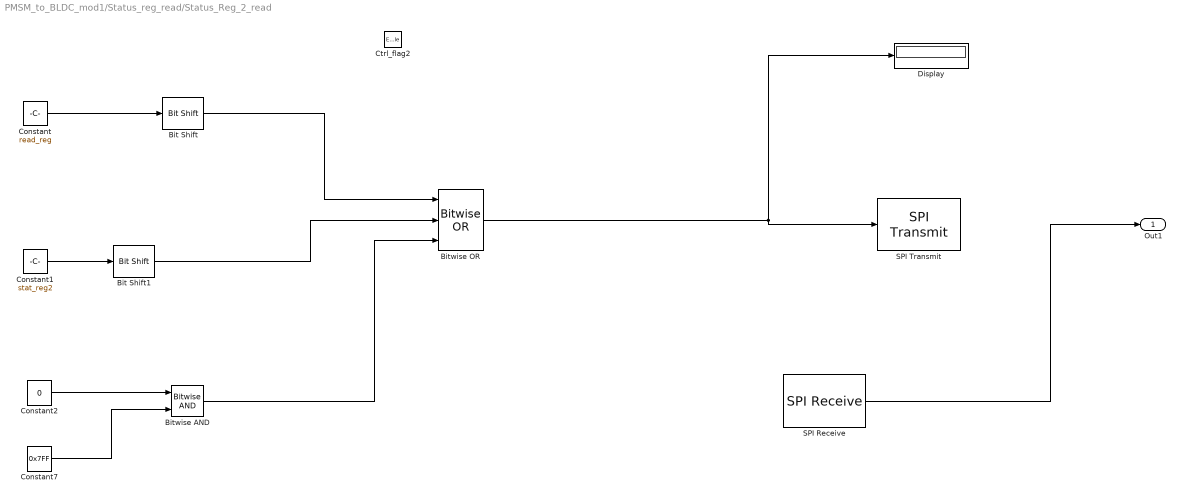
== system PMSM_to_BLDC_mod1/Status_reg_read/Status_Reg_2_read ==
  Ctrl_flag2 : EnablePort  StatesWhenEnabling=reset
  Bit Shift : hdlsllib/Logic and Bit Operations/Bit Shift  mode=Shift Left Logical  N=15
  Bit Shift1 : hdlsllib/Logic and Bit Operations/Bit Shift  mode=Shift Left Logical  N=11
  Bitwise AND : simulink/Logic and Bit Operations/Bitwise Operator  logicop=AND  UseBitMask=off  NumInputPorts=2  BitMask=bin2dec('11011001')  BitMaskRealWorld=Stored Integer
      settings: LibrarySourceBlock=|
      | simulink/Quick Insert/Logic and Bit
      | Operations/Bitwise AND
  Bitwise OR : simulink/Logic and Bit Operations/Bitwise Operator  logicop=OR  UseBitMask=off  NumInputPorts=3  BitMask=bin2dec('11011001')  BitMaskRealWorld=Stored Integer
      settings: LibrarySourceBlock=|
      | simulink/Quick Insert/Logic and Bit
      | Operations/Bitwise OR
  Constant : Constant  Value=read_reg  OutDataTypeStr=uint16
  Constant1 : Constant  Value=stat_reg2  OutDataTypeStr=uint16
  Constant2 : Constant  Value=0  OutDataTypeStr=uint16
  Constant7 : Constant  Value=0x7FF  OutDataTypeStr=uint16
  Display : Display
      settings: Format=hex (Stored Integer)
  SPI Receive : stm32blockslib/SPI Receive  SPIModuleSelect=SPI3  ClockPolarity=Low  ClockPhase=2 Edge  SPIModule=uint32(0)  Mode=Master  BusSpeed=uint32(1000000)  FirstBitToTransfer=Most significant bit (MSB)  ClockMode=0  BlockFunction=Read  EnableRegisterAddress=on  RegisterAddress=0  OutputDataType=uint8  OutputDataLength=15  OutputStatus=off  BlockingMode=on  Timeout=0.001  SampleTime=-1  DataBits=16  UseCustomSSPin=Explicit GPIO calls  ActiveLowSSPin=Active low  Port_Select=GPIOC  Pin=14
      settings: LibrarySourceBlock=stm32f4xxblockslib/SPI Receive
  SPI Transmit : stm32blockslib/SPI Transmit  SPIModuleSelect=SPI3  ClockPolarity=Low  ClockPhase=2 Edge  SPIModule=uint32(0)  Mode=Master  BusSpeed=uint32(1000000)  FirstBitToTransfer=Most significant bit (MSB)  ClockMode=0  BlockFunction=Write  EnableRegisterAddress=on  RegisterAddress=0  OutputDataType=uint8  OutputDataLength=1  OutputStatus=off  BlockingMode=on  Timeout=0.001  DataBits=16  UseCustomSSPin=Explicit GPIO calls  ActiveLowSSPin=Active low  Port_Select=GPIOC  Pin=14
      settings: LibrarySourceBlock=stm32f4xxblockslib/SPI Transmit
  Out1 : Outport  SampleTime=1  OutputWhenDisabled=reset  InitialOutput=[0]
  wires:
  Constant1/1 -> Bit Shift1/1
  Constant/1 -> Bit Shift/1
  Bit Shift/1 -> Bitwise OR/1
  Bit Shift1/1 -> Bitwise OR/2
  Constant2/1 -> Bitwise AND/1
  Constant7/1 -> Bitwise AND/2
  Bitwise AND/1 -> Bitwise OR/3
  Bitwise OR/1 -> SPI Transmit/1, Display/1
  SPI Receive/1 -> Out1/1

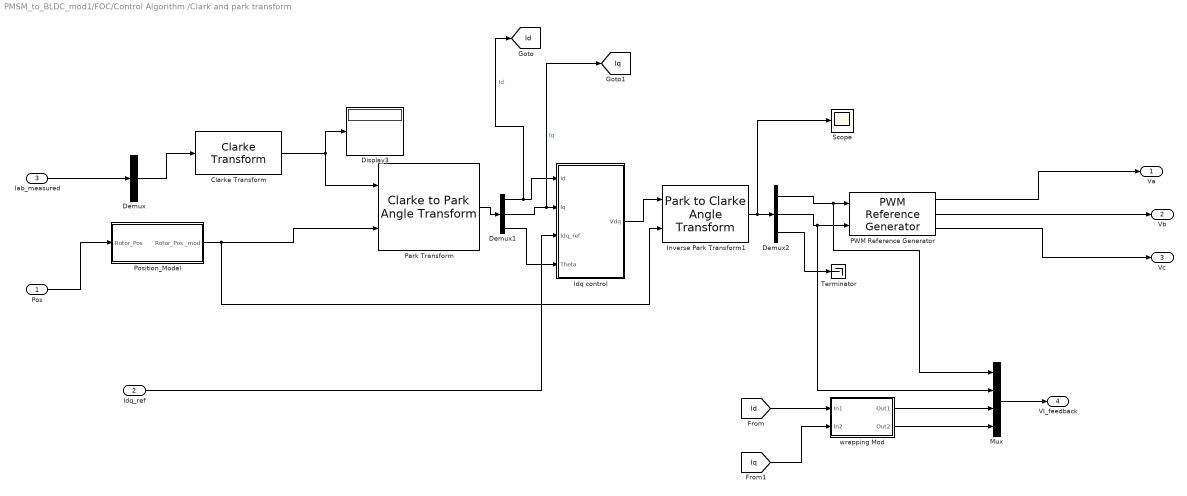
== system PMSM_to_BLDC_mod1/FOC/Control Algorithm /Clark and park transform ==
  Pos : Inport
  Idq_ref : Inport  Port=2
  Iab_measured : Inport  Port=3
  Clarke Transform : mcbeeMathTransformLib/Clarke Transform  VariantControl=Variant2  PowerInvariant=off  UseWithEmbedded=on  PhaseInput=Three inputs
      settings: LibrarySourceBlock=mcblib/Controls/Math Transforms/Clarke Transform
  Demux : Demux  Outputs=1
  Demux1 : Demux  Outputs=3
  Demux2 : Demux  Outputs=3
  Display3 : Display
  Idq control : Subsystem
  Inverse Park Transform1 : mcbeeMathTransformLib/Park to Clarke Angle Transform  AxisAlignment=D-axis  UseWithEmbedded=on  PhaseInput=Three inputs  ThetaInput=Electrical position  AngleInput=Radians  N_points=1024
      settings: LibrarySourceBlock=mcbhdllib/Controls/Math Transforms/Inverse Park Transform
  Mux : Mux
  PWM Reference Generator : mcbcontrolslib/PWM Reference Generator  inSignal=Valphabeta  modType=SVM: space vector modulation
      settings: LibrarySourceBlock=mcbhdllib/Controls/Math Transforms/PWM Reference Generator
  Park Transform : mcbeeMathTransformLib/Clarke to Park Angle Transform  AxisAlignment=D-axis  UseWithEmbedded=on  PhaseInput=Three inputs  ThetaInput=Electrical position  AngleInput=Radians  N_points=1024
      settings: LibrarySourceBlock=mcblib/Controls/Math Transforms/Park Transform
  Position_Model : Subsystem
  Scope : Scope
      settings: ActiveDisplayYMinimum=-1.6231207105132253  ActiveDisplayYMaximum=1.9168476700347847  DataLoggingVariableName=ScopeData9
  Terminator : Terminator
  wrapping Mod : Subsystem
  Va : Outport
  Vb : Outport  Port=2
  Vc : Outport  Port=3
  VI_feedback : Outport  Port=4
  tag scope: Id=global, Iq=global
  wires:
  Clarke Transform/1 -> Park Transform/1, Display3/1
  Demux/1 -> Clarke Transform/1
  PWM Reference Generator/1 -> Va/1
  PWM Reference Generator/2 -> Vb/1
  PWM Reference Generator/3 -> Vc/1
  Idq_ref/1 -> Idq control/3(Idq_ref)
  Mux/1 -> VI_feedback/1
  Iab_measured/1 -> Demux/1
  wrapping Mod/1(Out1) -> Mux/3
  wrapping Mod/2(Out2) -> Mux/4
  Pos/1 -> Position_Model/1(Rotor_Pos)
  Position_Model/1(Rotor_Pos _mod) -> Inverse Park Transform1/2, Park Transform/2
  Park Transform/1 -> Demux1/1
  Demux1/2 -> [Iq], Idq control/2(Iq)  "Iq"
  Demux1/3 -> Idq control/4(Theta)
  Idq control/1(Vdq) -> Inverse Park Transform1/1
  Inverse Park Transform1/1 -> Scope/1, Demux2/1
  Demux2/1 -> Mux/1, PWM Reference Generator/1
  Demux2/2 -> Mux/2, PWM Reference Generator/2
  Demux2/3 -> Terminator/1
  Demux1/1 -> [Id], Idq control/1(Id)  "Id"
  [Id] -> wrapping Mod/1(In1)
  [Iq] -> wrapping Mod/2(In2)

== system PMSM_to_BLDC_mod1/FOC/Control Algorithm /Speed & Iab handle ==
  VI_Feedback : Inport
  Iab_ADC : Inport  Port=2
  Data Type Conversion : DataTypeConversion  OutDataTypeStr=double  SaturateOnIntegerOverflow=off  RndMeth=Floor
  Phase current Mesurement : Subsystem
  Position and speed measurement : Subsystem
  POS : Outport
  Angular_Vel_Measured : Outport  Port=2
  Iab_measure : Outport  Port=3
  wires:
  VI_Feedback/1 -> Position and speed measurement/1(VI_feedback)
  Position and speed measurement/1(Pos) -> Data Type Conversion/1
  Position and speed measurement/2(Spd) -> Angular_Vel_Measured/1
  Iab_ADC/1 -> Phase current Mesurement/1(Iab_ADC)
  Phase current Mesurement/1(Iab) -> Iab_measure/1
  Data Type Conversion/1 -> POS/1

== system PMSM_to_BLDC_mod1/FOC/Control Algorithm /Subsystem1 ==
  Duty_cycle_raw : Inport
  Add : Sum
  Constant : Constant  Value=1.45
  Gain : Gain  Gain=1/3
  Duty Cycle : Outport
  wires:
  Constant/1 -> Add/2
  Add/1 -> Gain/1
  Duty_cycle_raw/1 -> Add/1
  Gain/1 -> Duty Cycle/1

== system PMSM_to_BLDC_mod1/FOC/Inverter/Simulation ==
  Gate_pulse : Inport
  Duty_cycle : Inport  Port=2
  Inverter&motor_Plant_model : Subsystem
  Scope : Scope  NumInputPorts=2
      settings: ActiveDisplayYMinimum=-223.34765299217423  ActiveDisplayYMaximum=224.46427656568537  DataLoggingVariableName=ScopeData7
  Simscape_Plantmodel : Subsystem
  Time Scope : Scope  Commented=on
      settings: TimeUnits=Metric (based on Time Span)  ActiveDisplayYMinimum=39.999999998732747  ActiveDisplayYMaximum=40.000000000141306  YLabel=Amplitude
  Phase_current : Outport
  wires:
  Inverter&motor_Plant_model/1(Electrical Pos) -> Scope/1  "Ele_Pos"
  Simscape_Plantmodel/1(Angular_vel_measured) -> Time Scope/1  "W_fb_sim"
  Inverter&motor_Plant_model/3(Motor_trq) -> Scope/2  "Motor_rpm"
  Inverter&motor_Plant_model/2(PhaseCurrent) -> Phase_current/1  "Phase_current"
  Gate_pulse/1 -> Simscape_Plantmodel/1(Duty Cycle_6pulse)
  Duty_cycle/1 -> Inverter&motor_Plant_model/1(Duty_cycle)

== system PMSM_to_BLDC_mod1/FOC/Inverter/Subsystem2 ==
  Duty cycle : Inport
  Demux : Demux  Outputs=3
  Demux1 : Demux  Outputs=3
  Gate_pulse : Scope  NumInputPorts=6
      settings: TimeUnits=Metric (based on Time Span)  ActiveDisplayYMinimum=-0.11142402829825793  ActiveDisplayYMaximum=1.1878033621780379  YLabel=Amplitude  DataLoggingVariableName=ScopeData10
  Mux : Mux  Inputs=6
  Subsystem : Subsystem
  Duty_cycle_6pulse : Outport
  wires:
  Demux1/1 -> Mux/2, Gate_pulse/4  "GA_L"
  Demux/2 -> Mux/3, Gate_pulse/2  "GB_H"
  Duty cycle/1 -> Demux/1, Subsystem/1(Duty Cycle)
  Demux/1 -> Mux/1, Gate_pulse/1  "GA_H"
  Subsystem/1(Gate_Lowside) -> Demux1/1
  Demux1/2 -> Mux/4, Gate_pulse/5  "GB_L"
  Demux1/3 -> Mux/6, Gate_pulse/6  "GC_L"
  Demux/3 -> Mux/5, Gate_pulse/3  "GC_H"
  Mux/1 -> Duty_cycle_6pulse/1

== system PMSM_to_BLDC_mod1/FOC/Speed_controls/Speed Control ==
  u : Inport
  PID Controller : slpidlib/PID Controller  Controller=PI  Form=Parallel  TimeDomain=Continuous-time  UseExternalTs=off  SampleTime=-1  IntegratorMethod=Forward Euler  FilterMethod=Forward Euler  ControllerParametersSource=internal  P=kp_speed  I=ki_speed*10/pwm_frequency  UseKiTs=on  D=0  UseExternalDerivativeSource=off  N=100  UseFilter=on  TunerSelectOption=Transfer Function Based (PID Tuner App)  InitialConditionSource=internal  InitialConditionForIntegrator=0  InitialConditionForFilter=0  DifferentiatorICPrevScaledInput=0  ExternalReset=none  TrackingMode=off  Kt=1  LimitOutput=off  SatLimitsSource=internal  UpperSaturationLimit=inf  LowerSaturationLimit=-inf  LinearizeAsGain=on  AntiWindupMode=none  Kb=1  LimitIntegrator=off  UpperIntegratorSaturationLimit=inf  LowerIntegratorSaturationLimit=-inf  POutMin=[]  POutMax=[]  IOutMin=[]  IOutMax=[]  DOutMin=[]  DOutMax=[]  NOutMin=[]  NOutMax=[]  SumOutMin=[]  SumOutMax=[]  SaturationOutMin=[]  SaturationOutMax=[]  PParamMin=[]  PParamMax=[]  IParamMin=[]  IParamMax=[]  DParamMin=[]  DParamMax=[]  NParamMin=[]  NParamMax=[]  KbParamMin=[]  KbParamMax=[]  KtParamMin=[]  KtParamMax=[]  KbOutMin=[]  KbOutMax=[]  KtOutMin=[]  KtOutMax=[]  IntegratorOutMin=[]  IntegratorOutMax=[]  FilterOutMin=[]  FilterOutMax=[]  SumI1OutMin=[]  SumI1OutMax=[]  SumI2OutMin=[]  SumI2OutMax=[]  SumI3OutMin=[]  SumI3OutMax=[]  SumI4OutMin=[]  SumI4OutMax=[]  SumDOutMin=[]  SumDOutMax=[]  DifferentiatorOutMin=[]  DifferentiatorOutMax=[]  FilterDiffOutCoefMin=[]  FilterDiffOutCoefMax=[]  ReciprocalOutMin=[]  ReciprocalOutMax=[]  SumDenOutMin=[]  SumDenOutMax=[]  SumNumOutMin=[]  SumNumOutMax=[]  DivideOutMin=[]  DivideOutMax=[]  UdiffTsProdOutMin=[]  UdiffTsProdOutMax=[]  NTsProdOutMin=[]  NTsProdOutMax=[]  UintegralTsProdOutMin=[]  UintegralTsProdOutMax=[]  UngainTsProdOutMin=[]  UngainTsProdOutMax=[]  ClampingZeroOutDataTypeStr=Inherit: Inherit via back propagation  ClampingZeroOutMin=[]  ClampingZeroOutMax=[]  FilterDenConstantOutDataTypeStr=Inherit: Inherit via back propagation  FilterDenConstantOutMin=[]  FilterDenConstantOutMax=[]  PCopyOutDataTypeStr=Inherit: Inherit via back propagation  PCopyOutMin=[]  PCopyOutMax=[]  NCopyOutDataTypeStr=Inherit: Inherit via back propagation  NCopyOutMin=[]  NCopyOutMax=[]  IntegratorContinuousStateAttributes=''  IntegratorStateMustResolveToSignalObject=off  IntegratorRTWStateStorageClass=Auto  FilterContinuousStateAttributes=''  FilterStateMustResolveToSignalObject=off  FilterRTWStateStorageClass=Auto  ParallelPVariant=InternalParameters  IdealPVariant=Disabled  IVariant=InternalParameters  DVariant=Disabled  IntegratorVariant=Continuous  SatVariant=Disabled  AWVariant=Passthrough  PCopyVariant=Disabled  TRVariant=Disabled  FdbkBlocksVariant=Forward  IdealPFdbkVariant=Disabled  SatFdbkVariant=Disabled  DerivativeFilterVariant=Disabled  NVariant=Disabled  NCopyVariant=Disabled_SignalSpec  FilterICVariant=Disabled  IntegratorICVariant=InternalICs  ExternalResetVariant=Disabled  TRSumVariant=Passthrough  SumFdbkVariant=Disabled  SumVariant=Sum_PI  TsampFilterVariant=InternalTs  TsampNgainVariant=Passthrough  TsampIntegralVariant=Disabled_SignalSpec  ExternalSaturationOutDataTypeStr=Inherit: Same as second input  DerivativeSourceVariant=Disabled  PreIntVariant=InternalPreInt
  Iq_ref : Outport
  wires:
  u/1 -> PID Controller/1
  PID Controller/1 -> Iq_ref/1

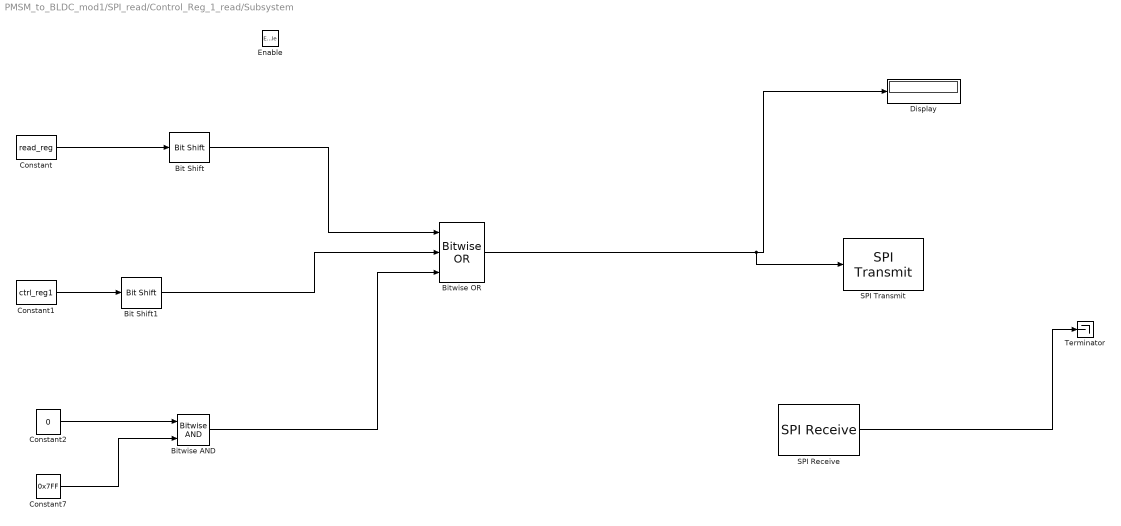
== system PMSM_to_BLDC_mod1/SPI_read/Control_Reg_1_read/Subsystem ==
  Enable : EnablePort  StatesWhenEnabling=reset
  Bit Shift : hdlsllib/Logic and Bit Operations/Bit Shift  mode=Shift Left Logical  N=15
  Bit Shift1 : hdlsllib/Logic and Bit Operations/Bit Shift  mode=Shift Left Logical  N=11
  Bitwise AND : simulink/Logic and Bit Operations/Bitwise Operator  logicop=AND  UseBitMask=off  NumInputPorts=2  BitMask=bin2dec('11011001')  BitMaskRealWorld=Stored Integer
      settings: LibrarySourceBlock=|
      | simulink/Quick Insert/Logic and Bit
      | Operations/Bitwise AND
  Bitwise OR : simulink/Logic and Bit Operations/Bitwise Operator  logicop=OR  UseBitMask=off  NumInputPorts=3  BitMask=bin2dec('11011001')  BitMaskRealWorld=Stored Integer
      settings: LibrarySourceBlock=|
      | simulink/Quick Insert/Logic and Bit
      | Operations/Bitwise OR
  Constant : Constant  Value=read_reg  OutDataTypeStr=uint16
  Constant1 : Constant  Value=ctrl_reg1  OutDataTypeStr=uint16
  Constant2 : Constant  Value=0  OutDataTypeStr=uint16
  Constant7 : Constant  Value=0x7FF  OutDataTypeStr=uint16
  Display : Display
      settings: Format=hex (Stored Integer)
  SPI Receive : stm32blockslib/SPI Receive  SPIModuleSelect=SPI3  ClockPolarity=Low  ClockPhase=2 Edge  SPIModule=uint32(0)  Mode=Master  BusSpeed=uint32(1000000)  FirstBitToTransfer=Most significant bit (MSB)  ClockMode=0  BlockFunction=Read  EnableRegisterAddress=on  RegisterAddress=0  OutputDataType=uint8  OutputDataLength=15  OutputStatus=off  BlockingMode=on  Timeout=0.001  SampleTime=-1  DataBits=16  UseCustomSSPin=Explicit GPIO calls  ActiveLowSSPin=Active low  Port_Select=GPIOC  Pin=14
      settings: LibrarySourceBlock=stm32f4xxblockslib/SPI Receive
  SPI Transmit : stm32blockslib/SPI Transmit  SPIModuleSelect=SPI3  ClockPolarity=Low  ClockPhase=2 Edge  SPIModule=uint32(0)  Mode=Master  BusSpeed=uint32(1000000)  FirstBitToTransfer=Most significant bit (MSB)  ClockMode=0  BlockFunction=Write  EnableRegisterAddress=on  RegisterAddress=0  OutputDataType=uint8  OutputDataLength=1  OutputStatus=off  BlockingMode=on  Timeout=0.001  DataBits=16  UseCustomSSPin=Explicit GPIO calls  ActiveLowSSPin=Active low  Port_Select=GPIOC  Pin=14
      settings: LibrarySourceBlock=stm32f4xxblockslib/SPI Transmit
  Terminator : Terminator
  wires:
  Bitwise OR/1 -> SPI Transmit/1, Display/1
  Constant2/1 -> Bitwise AND/1
  Bitwise AND/1 -> Bitwise OR/3
  Constant7/1 -> Bitwise AND/2
  Constant1/1 -> Bit Shift1/1
  Bit Shift/1 -> Bitwise OR/1
  Bit Shift1/1 -> Bitwise OR/2
  Constant/1 -> Bit Shift/1
  SPI Receive/1 -> Terminator/1

== system PMSM_to_BLDC_mod1/SPI_read/Control_Reg_1_read/Subsystem1 ==
  Ctrl_flag2 : EnablePort  StatesWhenEnabling=reset
  Constant : Constant  Value=0x9000
  SPI Receive : stm32blockslib/SPI Receive  SPIModuleSelect=SPI3  ClockPolarity=Low  ClockPhase=2 Edge  SPIModule=uint32(0)  Mode=Master  BusSpeed=uint32(1000000)  FirstBitToTransfer=Most significant bit (MSB)  ClockMode=0  BlockFunction=Read  EnableRegisterAddress=on  RegisterAddress=0  OutputDataType=uint8  OutputDataLength=1  OutputStatus=off  BlockingMode=on  Timeout=0.001  SampleTime=-1  DataBits=16  UseCustomSSPin=Explicit GPIO calls  ActiveLowSSPin=Active low  Port_Select=GPIOC  Pin=14
      settings: LibrarySourceBlock=stm32f4xxblockslib/SPI Receive
  SPI Transmit : stm32blockslib/SPI Transmit  SPIModuleSelect=SPI3  ClockPolarity=Low  ClockPhase=2 Edge  SPIModule=uint32(0)  Mode=Master  BusSpeed=uint32(1000000)  FirstBitToTransfer=Most significant bit (MSB)  ClockMode=0  BlockFunction=Write  EnableRegisterAddress=on  RegisterAddress=0  OutputDataType=uint8  OutputDataLength=1  OutputStatus=off  BlockingMode=on  Timeout=0.001  DataBits=16  UseCustomSSPin=Explicit GPIO calls  ActiveLowSSPin=Active low  Port_Select=GPIOC  Pin=14
      settings: LibrarySourceBlock=stm32f4xxblockslib/SPI Transmit
  Out1 : Outport  OutputWhenDisabled=reset  InitialOutput=[0]
  wires:
  Constant/1 -> SPI Transmit/1
  SPI Receive/1 -> Out1/1

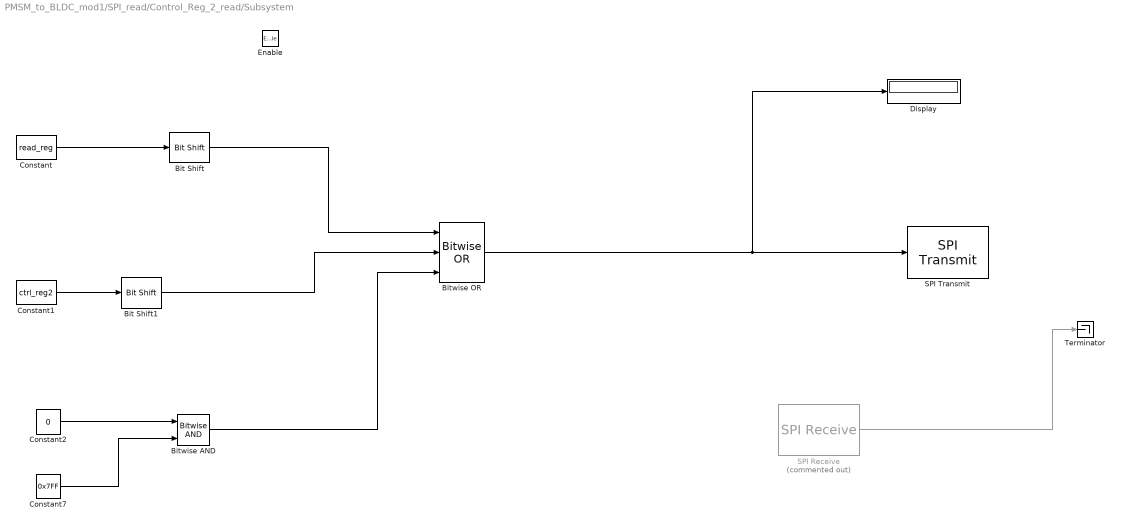
== system PMSM_to_BLDC_mod1/SPI_read/Control_Reg_2_read/Subsystem ==
  Enable : EnablePort  StatesWhenEnabling=reset
  Bit Shift : hdlsllib/Logic and Bit Operations/Bit Shift  mode=Shift Left Logical  N=15
  Bit Shift1 : hdlsllib/Logic and Bit Operations/Bit Shift  mode=Shift Left Logical  N=11
  Bitwise AND : simulink/Logic and Bit Operations/Bitwise Operator  logicop=AND  UseBitMask=off  NumInputPorts=2  BitMask=bin2dec('11011001')  BitMaskRealWorld=Stored Integer
      settings: LibrarySourceBlock=|
      | simulink/Quick Insert/Logic and Bit
      | Operations/Bitwise AND
  Bitwise OR : simulink/Logic and Bit Operations/Bitwise Operator  logicop=OR  UseBitMask=off  NumInputPorts=3  BitMask=bin2dec('11011001')  BitMaskRealWorld=Stored Integer
      settings: LibrarySourceBlock=|
      | simulink/Quick Insert/Logic and Bit
      | Operations/Bitwise OR
  Constant : Constant  Value=read_reg  OutDataTypeStr=uint16
  Constant1 : Constant  Value=ctrl_reg2  OutDataTypeStr=uint16
  Constant2 : Constant  Value=0  OutDataTypeStr=uint16
  Constant7 : Constant  Value=0x7FF  OutDataTypeStr=uint16
  Display : Display
      settings: Format=hex (Stored Integer)
  SPI Receive : stm32blockslib/SPI Receive  Commented=on  SPIModuleSelect=SPI3  ClockPolarity=Low  ClockPhase=2 Edge  SPIModule=uint32(0)  Mode=Master  BusSpeed=uint32(1000000)  FirstBitToTransfer=Most significant bit (MSB)  ClockMode=0  BlockFunction=Read  EnableRegisterAddress=on  RegisterAddress=0  OutputDataType=uint8  OutputDataLength=15  OutputStatus=off  BlockingMode=on  Timeout=0.001  SampleTime=-1  DataBits=16  UseCustomSSPin=Explicit GPIO calls  ActiveLowSSPin=Active low  Port_Select=GPIOC  Pin=14
      settings: LibrarySourceBlock=stm32f4xxblockslib/SPI Receive
  SPI Transmit : stm32blockslib/SPI Transmit  SPIModuleSelect=SPI3  ClockPolarity=Low  ClockPhase=2 Edge  SPIModule=uint32(0)  Mode=Master  BusSpeed=uint32(1000000)  FirstBitToTransfer=Most significant bit (MSB)  ClockMode=0  BlockFunction=Write  EnableRegisterAddress=on  RegisterAddress=0  OutputDataType=uint8  OutputDataLength=1  OutputStatus=off  BlockingMode=on  Timeout=0.001  DataBits=16  UseCustomSSPin=Explicit GPIO calls  ActiveLowSSPin=Active low  Port_Select=GPIOC  Pin=14
      settings: LibrarySourceBlock=stm32f4xxblockslib/SPI Transmit
  Terminator : Terminator
  wires:
  Bitwise OR/1 -> SPI Transmit/1, Display/1
  Constant2/1 -> Bitwise AND/1
  Bitwise AND/1 -> Bitwise OR/3
  Constant7/1 -> Bitwise AND/2
  Constant1/1 -> Bit Shift1/1
  Bit Shift/1 -> Bitwise OR/1
  Bit Shift1/1 -> Bitwise OR/2
  Constant/1 -> Bit Shift/1
  SPI Receive/1 -> Terminator/1

== system PMSM_to_BLDC_mod1/SPI_read/Control_Reg_2_read/Subsystem1 ==
  Enable : EnablePort  StatesWhenEnabling=reset
  Constant : Constant  Value=0X9800
  SPI Receive : stm32blockslib/SPI Receive  SPIModuleSelect=SPI3  ClockPolarity=Low  ClockPhase=2 Edge  SPIModule=uint32(0)  Mode=Master  BusSpeed=uint32(1000000)  FirstBitToTransfer=Most significant bit (MSB)  ClockMode=0  BlockFunction=Read  EnableRegisterAddress=on  RegisterAddress=0  OutputDataType=uint8  OutputDataLength=1  OutputStatus=off  BlockingMode=on  Timeout=0.001  SampleTime=-1  DataBits=16  UseCustomSSPin=Explicit GPIO calls  ActiveLowSSPin=Active low  Port_Select=GPIOC  Pin=14
      settings: LibrarySourceBlock=stm32f4xxblockslib/SPI Receive
  SPI Transmit : stm32blockslib/SPI Transmit  SPIModuleSelect=SPI3  ClockPolarity=Low  ClockPhase=2 Edge  SPIModule=uint32(0)  Mode=Master  BusSpeed=uint32(1000000)  FirstBitToTransfer=Most significant bit (MSB)  ClockMode=0  BlockFunction=Write  EnableRegisterAddress=on  RegisterAddress=0  OutputDataType=uint8  OutputDataLength=1  OutputStatus=off  BlockingMode=on  Timeout=0.001  DataBits=16  UseCustomSSPin=Explicit GPIO calls  ActiveLowSSPin=Active low  Port_Select=GPIOC  Pin=14
      settings: LibrarySourceBlock=stm32f4xxblockslib/SPI Transmit
  Out1 : Outport  OutputWhenDisabled=reset  InitialOutput=[0]
  wires:
  Constant/1 -> SPI Transmit/1
  SPI Receive/1 -> Out1/1

== system PMSM_to_BLDC_mod1/FOC/Control Algorithm /Clark and park transform/Idq control ==
  Id : Inport
  Iq : Inport  Port=2
  Idq_ref : Inport  Port=3
  Theta : Inport  Port=4
  Demux : Demux  Outputs=2
  Mux : Mux  Inputs=3
  PI Control for Iq : Subsystem
  PI control for Id : Subsystem
  Vdq : Outport
  wires:
  Idq_ref/1 -> Demux/1
  Id/1 -> PI control for Id/1(Inport)
  Iq/1 -> PI Control for Iq/1(Inport1)
  Demux/1 -> PI control for Id/2(In2)
  Demux/2 -> PI Control for Iq/2(In2)
  PI control for Id/1(y) -> Mux/1
  PI Control for Iq/1(y) -> Mux/2
  Mux/1 -> Vdq/1
  Theta/1 -> Mux/3

== system PMSM_to_BLDC_mod1/FOC/Control Algorithm /Clark and park transform/Position_Model ==
  Rotor_Pos : Inport
  Constant : Constant  Value=2*3.141
  Data Type Conversion1 : DataTypeConversion  OutDataTypeStr=double  ConvertRealWorld=Stored Integer (SI)  RndMeth=Floor
  Display : Display
  Mod : Math  Operator=mod
  Scope : Scope
      settings: ActiveDisplayYMinimum=-1  ActiveDisplayYMaximum=1  DataLoggingVariableName=ScopeData11
  Rotor_Pos _mod : Outport
  wires:
  Mod/1 -> Data Type Conversion1/1
  Constant/1 -> Mod/2
  Rotor_Pos/1 -> Scope/1, Mod/1  "Eps"
  Data Type Conversion1/1 -> Rotor_Pos _mod/1, Display/1

== system PMSM_to_BLDC_mod1/FOC/Control Algorithm /Clark and park transform/wrapping Mod ==
  In1 : Inport
  In2 : Inport  Port=2
  Constant1 : Constant  Value=2*3.141
  Data Type Conversion : DataTypeConversion  OutDataTypeStr=double  SaturateOnIntegerOverflow=off  RndMeth=Floor
  Data Type Conversion1 : DataTypeConversion  OutDataTypeStr=double  SaturateOnIntegerOverflow=off  RndMeth=Floor
  Mod1 : Math  Operator=mod
  Mod2 : Math  Operator=mod
  Out1 : Outport
  Out2 : Outport  Port=2
  wires:
  Constant1/1 -> Mod2/2, Mod1/2
  In1/1 -> Mod1/1
  In2/1 -> Mod2/1
  Mod2/1 -> Data Type Conversion1/1
  Mod1/1 -> Data Type Conversion/1
  Data Type Conversion/1 -> Out1/1
  Data Type Conversion1/1 -> Out2/1

== system PMSM_to_BLDC_mod1/FOC/Control Algorithm /Speed & Iab handle/Phase current Mesurement ==
  Iab_ADC : Inport
  Data Type Conversion : DataTypeConversion  SaturateOnIntegerOverflow=off  RndMeth=Floor
  Iab : Outport
  wires:
  Data Type Conversion/1 -> Iab/1
  Iab_ADC/1 -> Data Type Conversion/1
